simulink model "Modelo_final_sim"  (R2024b)
settings: Solver=FixedStepAuto  StartTime=0.0  StopTime=100  RelTol=1e-3  EnableMultiTasking=on
undefined symbols (not defined in the file): A, Ad, B, Bd, C, Cd, Dd, Discrete, K, Kr, Time, Ts
libraries: simulink x3, ctrlSharedLib x1
settings Model: CodeVerificationMode=processor-in-the-loop (pil)  ExtModeTrigDuration=2  Creator=alvar  LastModifiedBy=alvar
settings SolverCC: AutoInsertRateTranBlk=on
settings OptimizationCC: EnhancedBackFolding=on  PassReuseOutputArgsAs=Individual arguments  ZeroExternalMemoryAtStartup=off  ZeroInternalMemoryAtStartup=off  MaxStackSize=64  OptimizeBlockOrder=speed  DifferentSizesBufferReuse=on  OptimizationCustomize=off  EfficientTunableParamExpr=on
settings DebuggingCC: ParameterTunabilityLossMsg=error
settings HardwareCC: ProdBitPerInt=16  ProdBitPerPointer=16  ProdBitPerSizeT=16  ProdBitPerPtrDiffT=16  ProdLargestAtomicFloat=None  ProdWordSize=8  ProdHWDeviceType=Atmel->AVR
settings RTWCC: Description=Embedded Coder  SystemTargetFile=ert.tlc  HardwareBoard=Arduino Mega 2560  TemplateMakefile=ert_default_tmf  Toolchain=Arduino AVR  BuildConfiguration=Faster Runs
settings CodeAppCC: ForceParamTrailComments=on  IgnoreCustomStorageClasses=off  OperatorAnnotations=on  SimulinkDataObjDesc=on  SFDataObjDesc=on  InsertBlockDesc=on
settings ERTTargetCC: SupportContinuousTime=on  SupportNonInlinedSFcns=on  SupportVariableSizeSignals=on  ExtModeTransport=3  ExtModeStaticAlloc=on  ExtModeAutomaticAllocSize=off  ExtModeStaticAllocSize=2048  ExtModeMexFile=ext_xcp  ExtModeIntrfLevel=Level2 - Open  InlinedParameterPlacement=Hierarchical

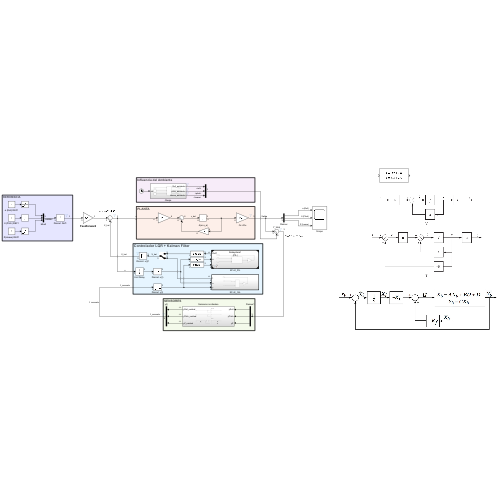
[thumbnail: Simulink's stored preview of the top-level diagram]
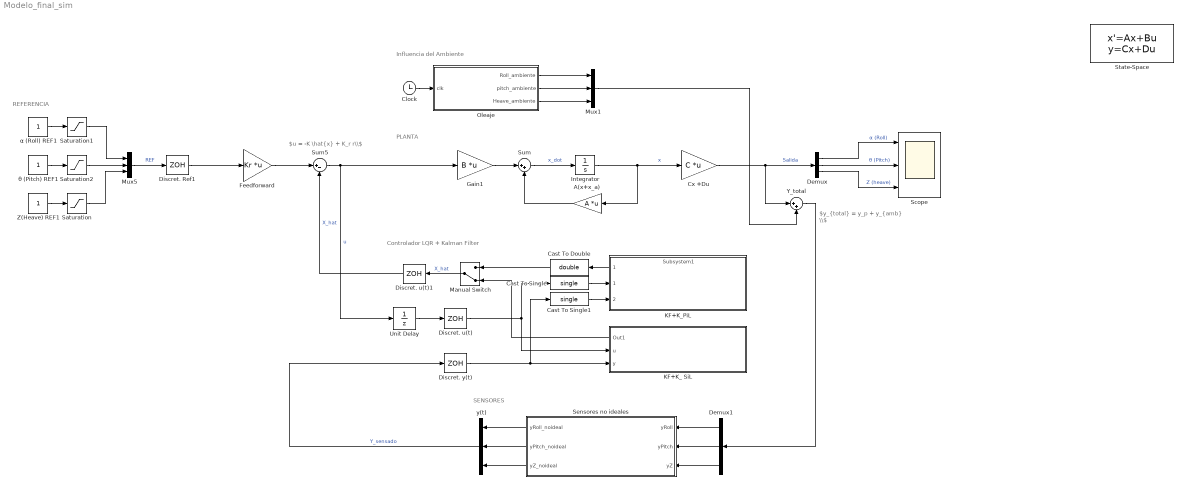
== system Modelo_final_sim ==
  note: Controlador LQR + Kalman Filter
  note: Influencia del Ambiente
  note: PLANTA
  note: SENSORES
  note: $u = -K \hat{x} + K_r r\\$
  note: REFERENCIA
  note: $y_{total} = y_p + y_{amb} \\$
  A(x+x_a) : Gain  Gain=A  Multiplication=Matrix(K*u)
  Cast To Double : DataTypeConversion  OutDataTypeStr=double  SaturateOnIntegerOverflow=off  RndMeth=Floor
  Cast To Single : DataTypeConversion  OutDataTypeStr=single  SaturateOnIntegerOverflow=off  RndMeth=Floor
  Cast To Single1 : DataTypeConversion  OutDataTypeStr=single  SaturateOnIntegerOverflow=off  RndMeth=Floor
  Clock : Clock
  Cx +Du : Gain  Gain=C  Multiplication=Matrix(K*u)
  Demux : Demux  Outputs=3
  Demux1 : Demux  Outputs=3
  Discret. Ref1 : ZeroOrderHold  SampleTime=Ts
  Discret. u(t) : ZeroOrderHold  SampleTime=Ts
  Discret. u(t)1 : ZeroOrderHold  SampleTime=Ts
  Discret. y(t) : ZeroOrderHold  SampleTime=Ts
  Feedforward : Gain  Gain=Kr  Multiplication=Matrix(K*u)
  Gain1 : Gain  Gain=B  Multiplication=Matrix(K*u)
  Integrator : Integrator
  KF+K_ SiL : Subsystem  TreatAsAtomicUnit=on
      settings: PortSchema="{\"entries\":[{\"content\":{\"sides\":[{\"content\":{\"connectorIds\":[\"Out1\",\"In1\",\"In2\"]},\"type\":\"ConnectorPlacement.EquallySpacedRectSide\",\"uuid\":\"cc2d612e-aa78-466d-8410-ff16b0e6f961\"},{\"content\":{\"side\":\"RIGHT\"},\"type\":\"ConnectorPlacement.EquallySpacedRectSide\",\"uuid\":\"817da510-bb6c-4ee0-9bb6-2ccb174f16ea\"},{\"content\":{\"side\":\"TOP\"},\"type\":\"ConnectorPlacement.EquallySpacedRectSide\",\"uuid\":\"e9a052d8-491e-466d-962f-48d8f048f36a\"}]},\"type\":\"ConnectorPlacement.EquallySpacedConnector\",\"uuid\":\"0f3e5d8d-280a-4078-bf61-ee03cd4f4d17\"}],\"packageUris\":[\"http://schema.mathworks.com/mf0/Connector/R2020b\"],\"version\":\"1.0\"}"
  KF+K_PiL : ModelReference  ModelNameDialog=Subsystem1.slx  SimulationMode=Processor-in-the-loop (PIL)  ModelReferenceVersion=1.22
      settings: PortSchema="{\"entries\":[{\"content\":{\"sides\":[{\"content\":{\"connectorIds\":[\"Out1\",\"In1\",\"In2\"]},\"type\":\"ConnectorPlacement.EquallySpacedRectSide\",\"uuid\":\"cc2d612e-aa78-466d-8410-ff16b0e6f961\"},{\"content\":{\"side\":\"RIGHT\"},\"type\":\"ConnectorPlacement.EquallySpacedRectSide\",\"uuid\":\"817da510-bb6c-4ee0-9bb6-2ccb174f16ea\"},{\"content\":{\"side\":\"TOP\"},\"type\":\"ConnectorPlacement.EquallySpacedRectSide\",\"uuid\":\"e9a052d8-491e-466d-962f-48d8f048f36a\"}]},\"type\":\"ConnectorPlacement.EquallySpacedConnector\",\"uuid\":\"0f3e5d8d-280a-4078-bf61-ee03cd4f4d17\"}],\"packageUris\":[\"http://schema.mathworks.com/mf0/Connector/R2020b\"],\"version\":\"1.0\"}"
  Manual Switch : ManualSwitch  CurrentSetting=0
  Mux1 : Mux  Inputs=3
  Mux5 : Mux  Inputs=3
  Oleaje : Subsystem
  Saturation : Saturate  UpperLimit=2  LowerLimit=1
  Saturation1 : Saturate  UpperLimit=90  LowerLimit=-90
  Saturation2 : Saturate  UpperLimit=90  LowerLimit=-90
  Scope : Scope  NumInputPorts=3
  Sensores no ideales : Subsystem
  State-Space : StateSpace  InitialCondition=0
  Sum : Sum  Inputs=|++
  Sum5 : Sum  Inputs=|+-
  Unit Delay : UnitDelay  SampleTime=Ts  HasFrameUpgradeWarning=on
  Y_total : Sum  Inputs=|++
  Z(Heave) REF1 : Constant
  y(t) : Mux  Inputs=3
  α (Roll) REF1 : Constant
  θ (Pitch) REF1 : Constant
  wires:
  Sum5/1 -> Gain1/1, Unit Delay/1  "u"
  Demux/3 -> Scope/3  "Z (heave)"
  Demux/2 -> Scope/2  "θ (Pitch)"
  Demux/1 -> Scope/1  "α (Roll)"
  Sensores no ideales/3(yZ_noideal) -> y(t)/3
  Demux1/3 -> Sensores no ideales/3(yZ)
  Sensores no ideales/2(yPitch_noideal) -> y(t)/2
  Demux1/1 -> Sensores no ideales/1(yRoll)
  Sensores no ideales/1(yRoll_noideal) -> y(t)/1
  Demux1/2 -> Sensores no ideales/2(yPitch)
  Cx +Du/1 -> Y_total/1, Demux/1  "Salida"
  Sum/1 -> Integrator/1  "x_dot"
  Gain1/1 -> Sum/1
  Oleaje/2(pitch_ambiente) -> Mux1/2
  Clock/1 -> Oleaje/1(clk)
  A(x+x_a)/1 -> Sum/2
  Y_total/1 -> Demux1/1
  Integrator/1 -> A(x+x_a)/1, Cx +Du/1  "x"
  Feedforward/1 -> Sum5/1
  y(t)/1 -> Discret. y(t)/1  "Y_sensado"
  Discret. u(t)1/1 -> Sum5/2  "X_hat"
  KF+K_ SiL/1(Out1) -> Manual Switch/2
  Cast To Double/1 -> Manual Switch/1
  Cast To Single/1 -> KF+K_PiL/1
  Unit Delay/1 -> Discret. u(t)/1
  Discret. u(t)/1 -> KF+K_ SiL/1(u), Cast To Single/1
  KF+K_PiL/1 -> Cast To Double/1
  Manual Switch/1 -> Discret. u(t)1/1  "X_hat"
  Discret. y(t)/1 -> Cast To Single1/1, KF+K_ SiL/2(y)
  Cast To Single1/1 -> KF+K_PiL/2
  θ (Pitch) REF1/1 -> Saturation2/1
  Saturation/1 -> Mux5/3
  Saturation1/1 -> Mux5/1
  α (Roll) REF1/1 -> Saturation1/1
  Mux5/1 -> Discret. Ref1/1  "REF"
  Z(Heave) REF1/1 -> Saturation/1
  Saturation2/1 -> Mux5/2
  Discret. Ref1/1 -> Feedforward/1
  Mux1/1 -> Y_total/2
  Oleaje/3(Heave_ambiente) -> Mux1/3
  Oleaje/1(Roll_ambiente) -> Mux1/1

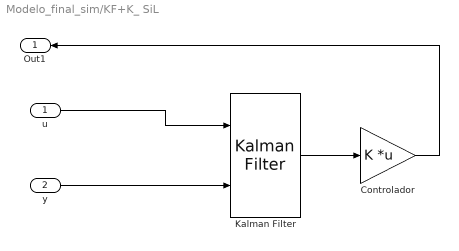
== system Modelo_final_sim/KF+K_ SiL ==
  u : Inport
  y : Inport  Port=2
  Controlador : Gain  Gain=K  Multiplication=Matrix(K*u)
  Kalman Filter : ctrlSharedLib/Kalman Filter  TimeDomain=Discrete-Time  UseCurrentEstimator=on  ModelSource=Individual A, B, C, D matrices  ModelSourceVariable=ss(0.95,1,1,0,1)  A=Ad  B=Bd  C=Cd  D=Dd  NumberOfStates=1  NumberOfInputs=1  NumberOfOutputs=1  InitialEstimateSource=Dialog  X0=0  P0=10  UseK=off  UseGH=off  NumberOfProcessNoiseInputs=1  G=1  TimeInvariantG=on  H=0  TimeInvariantH=on  Q=1e-18  TimeInvariantQ=on  R=0.003  TimeInvariantR=on  N=0  TimeInvariantN=on  AddInputPort=on  AddEnablePort=off  OutputEstimatedY=off  OutputP=off  Ts=Ts
  Out1 : Outport
  wires:
  Kalman Filter/1 -> Controlador/1
  u/1 -> Kalman Filter/1
  Controlador/1 -> Out1/1
  y/1 -> Kalman Filter/2

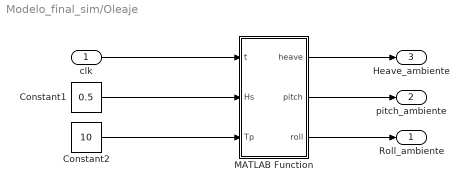
== system Modelo_final_sim/Oleaje ==
  clk : Inport
  Constant1 : Constant  Value=0.5
  Constant2 : Constant  Value=10
  MATLAB Function : MATLAB Function  TreatAsAtomicUnit=on
  Roll_ambiente : Outport
  pitch_ambiente : Outport  Port=2
  Heave_ambiente : Outport  Port=3
  wires:
  Constant1/1 -> MATLAB Function/2(Hs)
  clk/1 -> MATLAB Function/1(t)
  MATLAB Function/2(pitch) -> pitch_ambiente/1
  Constant2/1 -> MATLAB Function/3(Tp)
  MATLAB Function/3(roll) -> Roll_ambiente/1
  MATLAB Function/1(heave) -> Heave_ambiente/1

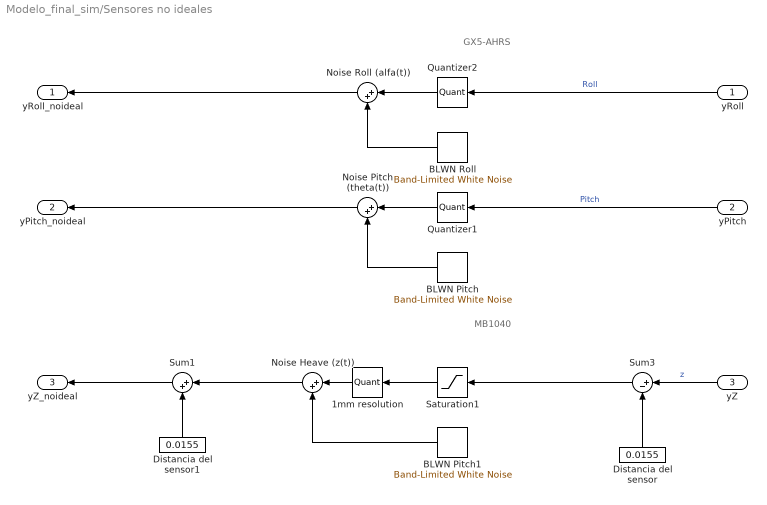
== system Modelo_final_sim/Sensores no ideales ==
  note: GX5-AHRS
  note: MB1040
  yRoll : Inport
  yPitch : Inport  Port=2
  yZ : Inport  Port=3
  1mm resolution : Quantizer  QuantizationInterval=0.001
  BLWN Pitch : simulink/Sources/Band-Limited White Noise  Cov=[0.0003]  Ts=0.01  seed=[23441]
  BLWN Pitch1 : simulink/Sources/Band-Limited White Noise  Cov=[0.0003]  Ts=0.01  seed=[23441]
  BLWN Roll : simulink/Sources/Band-Limited White Noise  Cov=[0.0003]  Ts=0.01  seed=[23341]
  Distancia del sensor : Constant  Value=0.0155
  Distancia del sensor1 : Constant  Value=0.0155
  Noise Heave (z(t)) : Sum  Inputs=|++
  Noise Pitch (theta(t)) : Sum  Inputs=|++
  Noise Roll (alfa(t)) : Sum  Inputs=|++
  Quantizer1 : Quantizer  QuantizationInterval=0.01
  Quantizer2 : Quantizer  QuantizationInterval=0.01
  Saturation1 : Saturate  UpperLimit=2  LowerLimit=0.0152
  Sum1 : Sum  Inputs=|++
  Sum3 : Sum  Inputs=|+-
  yRoll_noideal : Outport
  yPitch_noideal : Outport  Port=2
  yZ_noideal : Outport  Port=3
  wires:
  yZ/1 -> Sum3/1  "z"
  yPitch/1 -> Quantizer1/1  "Pitch"
  yRoll/1 -> Quantizer2/1  "Roll"
  Noise Roll (alfa(t))/1 -> yRoll_noideal/1
  Quantizer1/1 -> Noise Pitch (theta(t))/1
  BLWN Pitch/1 -> Noise Pitch (theta(t))/2
  Sum3/1 -> Saturation1/1
  Quantizer2/1 -> Noise Roll (alfa(t))/1
  BLWN Roll/1 -> Noise Roll (alfa(t))/2
  Distancia del sensor/1 -> Sum3/2
  Noise Pitch (theta(t))/1 -> yPitch_noideal/1
  Saturation1/1 -> 1mm resolution/1
  BLWN Pitch1/1 -> Noise Heave (z(t))/2
  1mm resolution/1 -> Noise Heave (z(t))/1
  Distancia del sensor1/1 -> Sum1/2
  Noise Heave (z(t))/1 -> Sum1/1
  Sum1/1 -> yZ_noideal/1

== matlab function Modelo_final_sim/Oleaje/MATLAB Function ==
  settings: updateMethod=DISCRETE
  data: t input; heave output; Hs input; Tp input; pitch output; roll output
function [heave, pitch, roll] = fcn(t, Hs, Tp)
%#codegen
% Esta función genera la elevación (heave), y los ángulos de inclinación 
% (pitch y roll) en el origen (0,0) para un oleaje P-M.
%
% Se utiliza t==0 para una inicialización robusta.

% -- Declaración de variables persistentes --
% Estas variables retienen su valor entre llamadas a la función.
persistent Anm fase omega kx ky

% -- Bloque de Inicialización --
% Este código se ejecuta UNA SOLA VEZ, al puro inicio de la simulación (t=0).
if t == 0
    
    % Parámetros fijos de la simulación
    N = 100;         % Número de componentes de frecuencia
    M = 50;          % Número de componentes de dirección
    g = 9.81;        % Aceleración de la gravedad

    % --- PRE-CÁLCULOS (se ejecutan solo una vez) ---
    fp = 1 / Tp;
    f_max = 4 * fp;
    df = f_max / N;
    f = df:df:f_max;
    omega = 2 * pi * f;

    d_theta = 2*pi / M;
    theta = d_theta:d_theta:2*pi;
    
    % Generar fases aleatorias (fijas para toda la simulación)
    fase = 2 * pi * rand(N, M);

    k_o = omega.^2 / g;
    kx = k_o' * cos(theta);
    ky = k_o' * sin(theta);
    
    A_pm = (5/16) * Hs^2 * fp^4;
    S = (A_pm ./ f.^5) .* exp(-1.25 * (fp^4 ./ f.^4));

    s = 10;
    D_theta = (2/pi) * (cos(theta/2)).^(2*s);
    D_theta(theta < -pi/2 | theta > pi/2) = 0;
    
    Anm = sqrt(2 * S' .* D_theta * df * d_theta);
end

% -- CÁLCULOS EN CADA PASO DE TIEMPO --
% Se requiere que las variables persistentes no estén vacías después de t=0
if isempty(Anm)
    % Si la inicialización no ha ocurrido (ej. si la simulación no empezó en t=0),
    % se asignan salidas cero para evitar errores.
    heave = 0;
    pitch = 0;
    roll = 0;
else
    % Cálculos normales para t > 0
    arg = -omega' * t + fase;
    heave = sum(Anm .* cos(arg), 'all');
    d_etadx = sum(Anm .* kx .* sin(arg), 'all');
    d_etady = sum(Anm .* ky .* sin(arg), 'all');
    pitch = atan(d_etadx);
    roll  = atan(d_etady);
end

end
